simulink model "speedgoat_test_SN5659_R2021b"  (R2021b)
settings: Solver=FixedStepDiscrete  StartTime=0.0  StopTime=inf  RelTol=1e-3
PreLoadFcn:
  | Ts_IO107 = 0.001;
  | Ts_IO107 = 0.001;
  | Ts_IO133 = 0.001
  | 
  | Ts_IO204 = 0.001;
  | 
  | 
  | Ts_IO503 = 0.01;
  | 
  | ts_IO612 = 1e-3;
  | Ts_IO682 = 0.005;
  | Ts_IO941 = 0.01;
InitFcn:
  | Ts_IO107 = 0.001;
  | Ts_IO107 = 0.001;
  | Ts_IO133 = 0.001
  | 
  | Ts_IO204 = 0.001;
  | 
  | 
  | Ts_IO503 = 0.01;
  | 
  | ts_IO612 = 1e-3;
  | Ts_IO682 = 0.005;
  | Ts_IO941 = 0.01;
StopFcn:
  | if isfile(['sdi_view_',bdroot,'.mldatx'])
  |  Simulink.sdi.clearPreferences();
  |  Simulink.sdi.view();
  |  pause(3);
  |  Simulink.sdi.loadView(['sdi_view_',bdroot,]);
  | end
undefined symbols (not defined in the file): C, IO682, standard
libraries: speedgoatlib_IO682 x161, simulink x49, slrealtimeseriallib x16, canmsglib x12, speedgoatlib_serial x9, speedgoatlib_IO612 x9, speedgoatlib_IO133 x5, speedgoatlib_IO107 x4, speedgoatlib_IO204 x3, speedgoatlib_IO421 x3, speedgoatlib_PIL x1
(part 1 of 4)
settings Model: Creator=yannick.orgas  LastModifiedBy=ACH
settings SolverCC: ConcurrentTasks=on  AlgebraicLoopSolver=TrustRegion  PositivePriorityOrder=on
settings DataIOCC: LimitDataPoints=on  SaveFormat=StructureWithTime
settings OptimizationCC: BlockReduction=off  OptimizeBlockIOStorage=off
settings DebuggingCC: TasksWithSamePriorityMsg=none  UnconnectedInputMsg=none  UnconnectedOutputMsg=none  UnconnectedLineMsg=none  SFMachineParentedDataDiag=warning
settings HardwareCC: ProdBitPerLong=64  ProdLongLongMode=on  ProdHWDeviceType=Intel->x86-64 (Linux 64)
settings RTWCC: Description=Simulink Real-Time  SystemTargetFile=slrealtime.tlc  TemplateMakefile=slrealtime_default_tmf  Toolchain=Simulink Real-Time Toolchain  BuildConfiguration=Faster Runs  CodeExecutionProfiling=on  TargetLang=C++
settings SimulinkRealTimeTargetCC: UseGCCFastMath=on

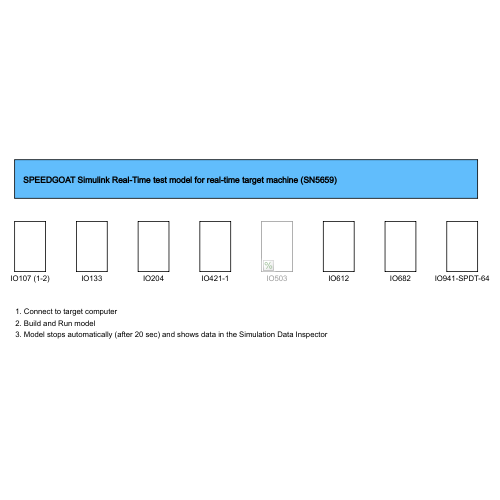
[thumbnail: Simulink's stored preview of the top-level diagram]
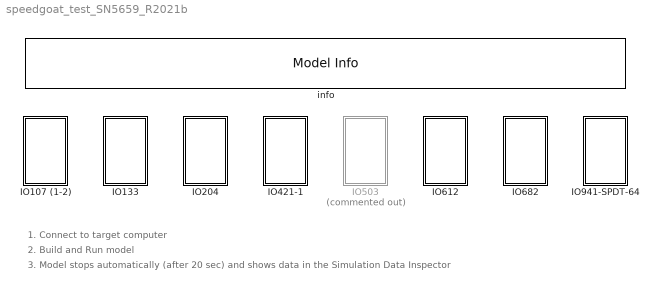
== system speedgoat_test_SN5659_R2021b ==
  note: 1. Connect to target computer
  note: 2. Build and Run model
  note: 3. Model stops automatically (after 20 sec) and shows data in the Simulation Data Inspector
  IO107 (1-2) : Subsystem
  IO133 : Subsystem
  IO204 : Subsystem
  IO421-1 : Subsystem
  IO503 : Subsystem  Commented=on
  IO612 : Subsystem
  IO682 : Subsystem
  IO941-SPDT-64 : Subsystem
  info : simulink/Model-Wide Utilities/Model Info  Frame=on  DisplayStringWithTags=SPEEDGOAT Simulink Real-Time test model for real-time target machine (SN5659)  HorizontalTextAlignment=Left  LeftAlignmentValue=0.02

== system speedgoat_test_SN5659_R2021b/IO107 (1-2) ==
  Analog output : speedgoatlib_IO107/Analog output  id=1  ts=-1  index=[1 2 3 4 5 6 7 8 9 10 11 12 13 14 15 16]  channels=[1 2 3 4 5 6 7 8 9 10 11 12 13 14 15 16]  range=1  pciSlot=-1
      settings: SourceProductName=Simulink Real-Time: Speedgoat Library
  Analog output1 : speedgoatlib_IO107/Analog output  id=2  ts=-1  index=[1 2 3 4 5 6 7 8 9 10 11 12 13 14 15 16]  channels=[1 2 3 4 5 6 7 8 9 10 11 12 13 14 15 16]  range=1  pciSlot=-1
      settings: SourceProductName=Simulink Real-Time: Speedgoat Library
  Setup : speedgoatlib_IO107/Setup  group=Analog output setup  id=1  range=+-10V  triggerSignal=TTL  groundSense=off  cal=on  pciSlot=-1  daChannel=[1:16]  daInitValue=[0]  daReset=[1]
      settings: SourceProductName=Simulink Real-Time: Speedgoat Library
  Setup1 : speedgoatlib_IO107/Setup  group=Module setup  id=2  range=+-10V  triggerSignal=TTL  groundSense=off  cal=on  pciSlot=-1  daChannel=[1:16]  daInitValue=[0]  daReset=[1]
      settings: SourceProductName=Simulink Real-Time: Speedgoat Library
  Sine Wave : Sin  Amplitude=10  Frequency=2*pi*50  SampleTime=Ts_IO107
  Sine Wave1 : Sin  Amplitude=10  Frequency=2*pi*50  SampleTime=Ts_IO107
  wires:
  Sine Wave/1 -> Analog output/1, Analog output/2, Analog output/3, Analog output/4, Analog output/5, Analog output/6, Analog output/7, Analog output/8, Analog output/9, Analog output/10, Analog output/11, Analog output/12, Analog output/13, Analog output/14, Analog output/15, Analog output/16
  Sine Wave1/1 -> Analog output1/1, Analog output1/2, Analog output1/3, Analog output1/4, Analog output1/5, Analog output1/6, Analog output1/7, Analog output1/8, Analog output1/9, Analog output1/10, Analog output1/11, Analog output1/12, Analog output1/13, Analog output1/14, Analog output1/15, Analog output1/16

== system speedgoat_test_SN5659_R2021b/IO133 ==
  "Analog input v2 " : speedgoatlib_IO133/Analog input v2   parModuleId=1  parSampleTime=Ts_IO133  parPciSlot=-1  parAdcChannels=[1 2 3 4]  parAdcVoltageRange=[2 2]  parAdcOversamplRate=[1 1]  parAdcContSampling=0  parAdcDmaEnable=0  parAdcActiveDmaDevices=[1 1]  parAdcFrameSize=100
      settings: SourceProductName=Simulink Real-Time: Speedgoat I/O Driver Library
  "Analog output v2 " : speedgoatlib_IO133/Analog output v2   parModuleId=1  parSampleTime=Ts_IO133  parPciSlot=-1  parDacChannels=[1 2 3 4]  parDacVoltageRange=[4 4 6 6 5 5 5 5]  parDacInitValues=[0 0 0 0]  parDacReset=[1 1 1 1]  parDacSyncOut=1  parDacDmaEnable=0  parDacActiveDmaDevices=[1 1]  parDacDmaLatency=2  parDacFrameSize=100
      settings: SourceProductName=Simulink Real-Time: Speedgoat I/O Driver Library
  "Digital input v2 " : speedgoatlib_IO133/Digital input v2   parModuleId=1  parSampleTime=Ts_IO133  parPciSlot=-1  parDiChannels=[8 9]
      settings: SourceProductName=Simulink Real-Time: Speedgoat I/O Driver Library
  "Digital output v2 " : speedgoatlib_IO133/Digital output v2   parModuleId=1  parSampleTime=Ts_IO133  parPciSlot=-1  parDoChannels=[1 2]  parDoInitValues=[0 0]  parDoReset=[1 1]
      settings: SourceProductName=Simulink Real-Time: Speedgoat I/O Driver Library
  Gain : Gain  Gain=2
  Gain1 : Gain  Gain=4
  Gain2 : Gain  Gain=6
  Gain3 : Gain  Gain=8
  Pulse Generator : DiscretePulseGenerator  Period=20  PulseWidth=5  SampleTime=Ts_IO133
  Pulse Generator1 : DiscretePulseGenerator  Period=20  PulseWidth=10  SampleTime=Ts_IO133
  "Scope 2 " : Scope  NumInputPorts=4
  "Scope 4 " : Scope  NumInputPorts=2
  "Setup v2 " : speedgoatlib_IO133/Setup v2   parPciSlot=-1  parModuleId=1  parInterModuleSync=None  parConvClockBaseRate=20MHz  parConvClock1Divider=20000  parConvClock2Divider=20000  parFrameTriggerEnable=off  parFrameTriggerDivider=10  parConvClock1BaseRate=1  parConvClock2BaseRate=1  parFrameTriggerClock=1  parAdcChannels=1:4  parAdcRange1=+-10V  parAdcRange2=+-10V  parAdcVoltageRange=[2 2]  parAdcOversampling1=None  parAdcOversampling2=None  parAdcOversamplRate=[1 1]  parAdcAutoCorrection=on  parAdcContSampling=off  parAdcDmaEnable=off  parAdcDmaClock=Clock 1  parAdcFrameSize_=100  parAdcSampleTime_=-1  parAdcActiveDmaDevices=[1 1]  parAdcFrameTriggerEnable=0  parAdcFrameSize=100  parAdcSampleTime=0.1  parDacChannels=1:4  parDacInitValues=0  parDacReset=1  parDacRange1=+-5V  parDacRange2=+-5V  parDacRange3=+-10.8V  parDacRange4=+-10.8V  parDacRange5=+-10V  parDacRange6=+-10V  parDacRange7=+-10V  parDacRange8=+-10V  parDacVoltageRange=[4 4 6 6 5 5 5 5]  parDacAutoCorrection=on  parDacSyncOut=on  parDacDmaEnable=off  parDacDmaLatency=Until next frame  parDacDmaClock=Clock 1  parDacFrameSize_=100  parDacSampleTime_=-1  parDacActiveDmaDevices=[1 1]  parDacFrameTriggerEnable=0  parDacFrameSize=100  parDacSampleTime=0.1  parDoChannels=1:2  parDoInitValues=0  parDoReset=1  parDiChannels=8:9  parDiDebounceEnable=off  parDiDebounceTime=0  parDiDebounceValue=0  parDioPullRefFront=Pull-up 3.3V  parDioPullRefRear=Floating
      settings: SourceProductName=Simulink Real-Time: Speedgoat I/O Driver Library
  Sine Wave : Sin  Frequency=50  SampleTime=0
  wires:
  Pulse Generator/1 -> "Digital output v2 "/1
  Gain1/1 -> "Analog output v2 "/2
  Gain/1 -> "Analog output v2 "/1
  Gain3/1 -> "Analog output v2 "/4
  Gain2/1 -> "Analog output v2 "/3
  Sine Wave/1 -> Gain/1, Gain1/1, Gain2/1, Gain3/1
  Pulse Generator1/1 -> "Digital output v2 "/2
  "Analog input v2 "/1 -> "Scope 2 "/1  "IO133_AI_CH1"
  "Analog input v2 "/2 -> "Scope 2 "/2  "IO133_AI_CH2"
  "Analog input v2 "/3 -> "Scope 2 "/3  "IO133_AI_CH3"
  "Analog input v2 "/4 -> "Scope 2 "/4  "IO133_AI_CH4"
  "Digital input v2 "/1 -> "Scope 4 "/1  "IO133_DI_CH8"
  "Digital input v2 "/2 -> "Scope 4 "/2  "IO133_DI_CH9"

== system speedgoat_test_SN5659_R2021b/IO204 ==
  Gain : Gain  Gain=2
  Gain1 : Gain  Gain=3
  Gain2 : Gain  Gain=4
  Pulse Generator : DiscretePulseGenerator  Period=20  PulseWidth=10  SampleTime=Ts_IO204
  Read : speedgoatlib_IO204/Read  id=1  group=Input  portType=16 ports of type double  ts=Ts_IO204  pciSlot=-1
      settings: SourceProductName=Simulink Real-Time: Speedgoat Library
  "Scope (xPC) " : Scope  NumInputPorts=4
  Setup : speedgoatlib_IO204/Setup  group=Module setup  id=1  pciSlot=-1  debounceEnable=on  debounceValue=0.001/10  reset=[0]  value=[0]
      settings: SourceProductName=Simulink Real-Time: Speedgoat Library
  Write : speedgoatlib_IO204/Write  id=1  portType=16 ports of type double  ts=-1  pciSlot=-1
      settings: SourceProductName=Simulink Real-Time: Speedgoat Library
  wires:
  Pulse Generator/1 -> Write/16, Write/11, Write/6, Write/1
  Read/6 -> Gain/1
  Read/11 -> Gain1/1
  Read/16 -> Gain2/1
  Read/1 -> "Scope (xPC) "/1  "IO204_CH1"
  Gain/1 -> "Scope (xPC) "/2  "IO204_CH6"
  Gain1/1 -> "Scope (xPC) "/3  "IO204_CH11"
  Gain2/1 -> "Scope (xPC) "/4  "IO204_CH16"

== system speedgoat_test_SN5659_R2021b/IO421-1 ==
  LVDT read : speedgoatlib_IO421/LVDT//RVDT/LVDT read  id=1  slot=1  channels=1  wiring=0  expectedVLL=7.0711  expectedVREF=18.3848  ts=0.001  pciSlot=-1
      settings: SourceProductName=Simulink Real-Time: Speedgoat Library
  LVDT read1 : speedgoatlib_IO421/LVDT//RVDT/LVDT read  id=1  slot=2  channels=1  wiring=0  expectedVLL=7.0711  expectedVREF=18.3848  ts=0.001  pciSlot=-1
      settings: SourceProductName=Simulink Real-Time: Speedgoat Library
  REF : speedgoatlib_IO421/W/REF  id=1  slot=3  frequency=47  voltage=26/sqrt(2)  pciSlot=-1
      settings: SourceProductName=Simulink Real-Time: Speedgoat I/O Blockset
  "Scope  " : Scope
  Scope  1 : Scope
  wires:
  LVDT read/1 -> "Scope  "/1  "IO421_LVDT_POS(1)"
  LVDT read1/1 -> Scope  1/1  "IO421_LVDT_POS(2)"

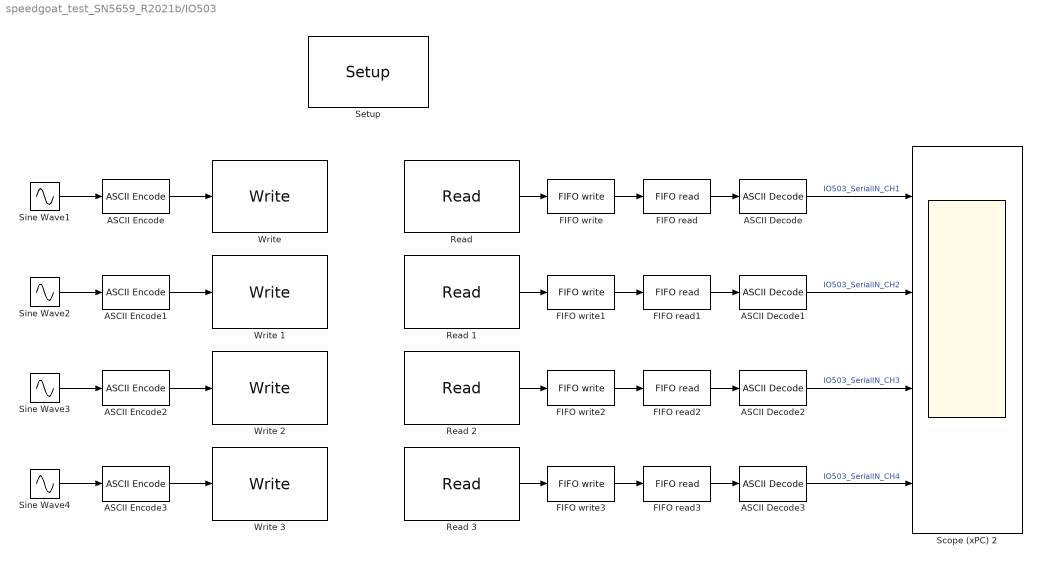
== system speedgoat_test_SN5659_R2021b/IO503 ==
  ASCII Decode{,1..3} (4 alike) : slrealtimeseriallib/ASCII Decode  format=%f\r  nvars=1  vartypes={'double'}
      settings: SourceProductBaseCode=XP
  ASCII Encode{,1..3} (4 alike) : slrealtimeseriallib/ASCII Encode  format=%f\r  nvars=1  maxlength=64  vartypes={ 'double' }
      settings: SourceProductBaseCode=XP
  FIFO read{,1..3} (4 alike) : slrealtimeseriallib/FIFO read  maxsize=64  minsize=1  usedelimiter=on  delimiter=13  outputtype=8 bit uint null terminated  enable=off  enableout=off  sampletime=Ts_IO503
      settings: SourceProductBaseCode=XP
  FIFO write : slrealtimeseriallib/FIFO write  size=64  inputtype=count+32 bit uint  present=off  sampletime=-1  id=Rx Ch1 overflow
      settings: SourceProductBaseCode=XP
  FIFO write1 : slrealtimeseriallib/FIFO write  size=64  inputtype=count+32 bit uint  present=off  sampletime=-1  id=Rx Ch2 overflow
      settings: SourceProductBaseCode=XP
  FIFO write2 : slrealtimeseriallib/FIFO write  size=64  inputtype=count+32 bit uint  present=off  sampletime=-1  id=Rx Ch3 overflow
      settings: SourceProductBaseCode=XP
  FIFO write3 : slrealtimeseriallib/FIFO write  size=64  inputtype=count+32 bit uint  present=off  sampletime=-1  id=Rx Ch4 overflow
      settings: SourceProductBaseCode=XP
  "Read " : speedgoatlib_serial/Speedgoat Shared blocks/Read   parModuleType=IO503  parModuleId=1  parChannel=1  parSampleTime=Ts_IO503  parFlush=on  parEnLegacy=on  parDataType=count+32 bit uint  parSlot=-1  parRxSwFifoSize=64
  Read 1 : speedgoatlib_serial/Speedgoat Shared blocks/Read   parModuleType=IO503  parModuleId=1  parChannel=2  parSampleTime=Ts_IO503  parFlush=on  parEnLegacy=on  parDataType=count+32 bit uint  parSlot=-1  parRxSwFifoSize=64
  Read 2 : speedgoatlib_serial/Speedgoat Shared blocks/Read   parModuleType=IO503  parModuleId=1  parChannel=3  parSampleTime=Ts_IO503  parFlush=on  parEnLegacy=on  parDataType=count+32 bit uint  parSlot=-1  parRxSwFifoSize=64
  Read 3 : speedgoatlib_serial/Speedgoat Shared blocks/Read   parModuleType=IO503  parModuleId=1  parChannel=4  parSampleTime=Ts_IO503  parFlush=on  parEnLegacy=on  parDataType=count+32 bit uint  parSlot=-1  parRxSwFifoSize=64
  "Scope (xPC) 2 " : Scope  NumInputPorts=4
  "Setup " : speedgoatlib_serial/Speedgoat Shared blocks/Setup   parModuleType=IO503  parModuleId=1  parSlot=-1  parTransceiver1=RS232  parTransceiver2=RS232  parTransceiver3=RS422  parTransceiver4=RS422  parTransceiver5=RS232  parTransceiver6=RS232  parTransceiver7=RS232  parTransceiver8=RS232  parTxTerm1=off  parRxTerm1=off  parMessageMonitoring1=off  parAutoTurnaround1=off  parTurnaroundDelay1=0  parStandardBaud1=on  parBaudrate1=921600  parBaudDivisor1=1  parSamplingRate1=16x (standard)  parPrescale1=off  parCalcBaud1=2764800  parParity1=None  parDataBits1=8  parStopBits1=1  parTxTrigLvl1=1  parRxTrigLvl1=8  parHandshake1=none  parRtsHysteresis1=0  parXon1=17  parXoff1=19  parTxSwFifoSize1=64  parRxSwFifoSize1=64  parTxTerm2=off  parRxTerm2=off  parMessageMonitoring2=off  parAutoTurnaround2=off  parTurnaroundDelay2=0  parStandardBaud2=on  parBaudrate2=921600  parBaudDivisor2=1  parSamplingRate2=16x (standard)  parPrescale2=off  parCalcBaud2=2764800  parParity2=None  parDataBits2=8  parStopBits2=1  parTxTrigLvl2=1  parRxTrigLvl2=8  parHandshake2=none  parRtsHysteresis2=0  parXon2=17  parXoff2=19  parTxSwFifoSize2=64  parRxSwFifoSize2=64  parTxTerm3=off  parRxTerm3=on  parMessageMonitoring3=off  parAutoTurnaround3=off  parTurnaroundDelay3=0  parStandardBaud3=on  parBaudrate3=2764800  parBaudDivisor3=1  parSamplingRate3=16x (standard)  parPrescale3=off  parCalcBaud3=2764800  parParity3=None  parDataBits3=8  parStopBits3=1  parTxTrigLvl3=1  parRxTrigLvl3=8  parHandshake3=none  parRtsHysteresis3=0  parXon3=17  parXoff3=19  parTxSwFifoSize3=64  parRxSwFifoSize3=64  parTxTerm4=off  parRxTerm4=on  parMessageMonitoring4=off  parAutoTurnaround4=off  parTurnaroundDelay4=0  parStandardBaud4=on  parBaudrate4=2764800  parBaudDivisor4=1  parSamplingRate4=16x (standard)  parPrescale4=off  parCalcBaud4=2764800  parParity4=None  parDataBits4=8  parStopBits4=1  parTxTrigLvl4=1  parRxTrigLvl4=8  parHandshake4=none  parRtsHysteresis4=0  parXon4=17  parXoff4=19  parTxSwFifoSize4=64  parRxSwFifoSize4=64  parTxTerm5=off  parRxTerm5=off  parMessageMonitoring5=off  parAutoTurnaround5=off  parTurnaroundDelay5=0  parStandardBaud5=on  parBaudrate5=115200  parBaudDivisor5=1  parSamplingRate5=16x (standard)  parPrescale5=off  parCalcBaud5=2764800  parParity5=None  parDataBits5=8  parStopBits5=1  parTxTrigLvl5=1  parRxTrigLvl5=1  parHandshake5=none  parRtsHysteresis5=0  parXon5=17  parXoff5=19  parTxSwFifoSize5=1024  parRxSwFifoSize5=1024  parTxTerm6=off  parRxTerm6=off  parMessageMonitoring6=off  parAutoTurnaround6=off  parTurnaroundDelay6=0  parStandardBaud6=on  parBaudrate6=115200  parBaudDivisor6=1  parSamplingRate6=16x (standard)  parPrescale6=off  parCalcBaud6=2764800  parParity6=None  parDataBits6=8  parStopBits6=1  parTxTrigLvl6=1  parRxTrigLvl6=1  parHandshake6=none  parRtsHysteresis6=0  parXon6=17  parXoff6=19  parTxSwFifoSize6=1024  parRxSwFifoSize6=1024  parTxTerm7=off  parRxTerm7=off  parMessageMonitoring7=off  parAutoTurnaround7=off  parTurnaroundDelay7=0  parStandardBaud7=on  parBaudrate7=115200  parBaudDivisor7=1  parSamplingRate7=16x (standard)  parPrescale7=off  parCalcBaud7=2764800  parParity7=None  parDataBits7=8  parStopBits7=1  parTxTrigLvl7=1  parRxTrigLvl7=1  parHandshake7=none  parRtsHysteresis7=0  parXon7=17  parXoff7=19  parTxSwFifoSize7=1024  parRxSwFifoSize7=1024  parTxTerm8=off  parRxTerm8=off  parMessageMonitoring8=off  parAutoTurnaround8=off  parTurnaroundDelay8=0  parStandardBaud8=on  parBaudrate8=115200  parBaudDivisor8=1  parSamplingRate8=16x (standard)  parPrescale8=off  parCalcBaud8=2764800  parParity8=None  parDataBits8=8  parStopBits8=1  parTxTrigLvl8=1  parRxTrigLvl8=1  parHandshake8=none  parRtsHysteresis8=0  parXon8=17  parXoff8=19  parTxSwFifoSize8=1024  parRxSwFifoSize8=1024
      settings: SourceProductName=Simulink Real-Time: Speedgoat I/O Driver Library
  Sine Wave1 : Sin  Amplitude=10  Bias=127  Frequency=1*2*pi  SampleTime=Ts_IO503
  Sine Wave2 : Sin  Amplitude=20  Bias=127  Frequency=1*2*pi  SampleTime=Ts_IO503
  Sine Wave3 : Sin  Amplitude=30  Bias=127  Frequency=1*2*pi  SampleTime=Ts_IO503
  Sine Wave4 : Sin  Amplitude=40  Bias=127  Frequency=1*2*pi  SampleTime=Ts_IO503
  "Write " : speedgoatlib_serial/Speedgoat Shared blocks/Write   parModuleType=IO503  parModuleId=1  parChannel=1  parSampleTime=-1  parEnLegacy=on  parDataType=8 bit uint null terminated  parSlot=-1  parTxSwFifoSize=64
  Write 1 : speedgoatlib_serial/Speedgoat Shared blocks/Write   parModuleType=IO503  parModuleId=1  parChannel=2  parSampleTime=-1  parEnLegacy=on  parDataType=8 bit uint null terminated  parSlot=-1  parTxSwFifoSize=64
  Write 2 : speedgoatlib_serial/Speedgoat Shared blocks/Write   parModuleType=IO503  parModuleId=1  parChannel=3  parSampleTime=-1  parEnLegacy=on  parDataType=8 bit uint null terminated  parSlot=-1  parTxSwFifoSize=64
  Write 3 : speedgoatlib_serial/Speedgoat Shared blocks/Write   parModuleType=IO503  parModuleId=1  parChannel=4  parSampleTime=-1  parEnLegacy=on  parDataType=8 bit uint null terminated  parSlot=-1  parTxSwFifoSize=64
  wires:
  Sine Wave4/1 -> ASCII Encode3/1
  Sine Wave3/1 -> ASCII Encode2/1
  Sine Wave1/1 -> ASCII Encode/1
  Sine Wave2/1 -> ASCII Encode1/1
  ASCII Decode/1 -> "Scope (xPC) 2 "/1  "IO503_SerialIN_CH1"
  ASCII Decode1/1 -> "Scope (xPC) 2 "/2  "IO503_SerialIN_CH2"
  ASCII Decode2/1 -> "Scope (xPC) 2 "/3  "IO503_SerialIN_CH3"
  ASCII Decode3/1 -> "Scope (xPC) 2 "/4  "IO503_SerialIN_CH4"
  FIFO write/1 -> FIFO read/1
  "Read "/1 -> FIFO write/1
  FIFO write1/1 -> FIFO read1/1
  Read 1/1 -> FIFO write1/1
  FIFO write2/1 -> FIFO read2/1
  FIFO write3/1 -> FIFO read3/1
  FIFO read1/1 -> ASCII Decode1/1
  FIFO read2/1 -> ASCII Decode2/1
  FIFO read3/1 -> ASCII Decode3/1
  Read 2/1 -> FIFO write2/1
  Read 3/1 -> FIFO write3/1
  ASCII Encode/1 -> "Write "/1
  FIFO read/1 -> ASCII Decode/1
  ASCII Encode1/1 -> Write 1/1
  ASCII Encode2/1 -> Write 2/1
  ASCII Encode3/1 -> Write 3/1

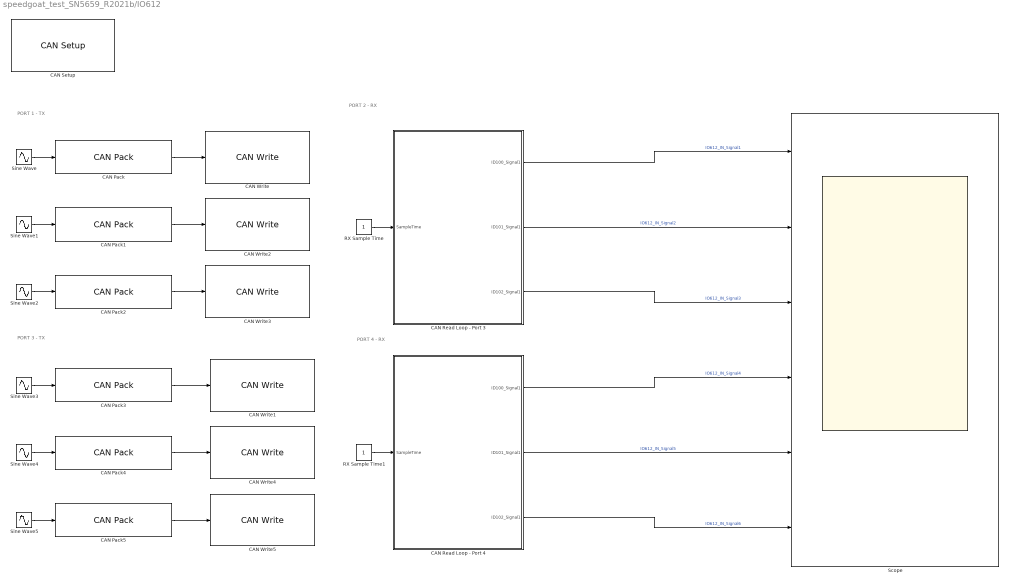
== system speedgoat_test_SN5659_R2021b/IO612 ==
  note: PORT 4 - RX
  note: PORT 1 - TX
  note: PORT 3 - TX
  note: PORT 2 - RX
  CAN Pack : canmsglib/CAN Pack  MsgList=(none)  MsgName=CAN Msg  MsgIDType=Standard (11-bit identifier)  MsgIdentifier=100  MsgLength=8  Remote=off  ApplyMinMax=off  BusOutput=off  SignalInfo={'Signal1','0','64','LE','double','Standard','0','1','0','-Inf','Inf'}
      settings: SourceProductBaseCode=ME,XP,VN  DataFormat=manually specified signals
  CAN Pack1 : canmsglib/CAN Pack  MsgList=(none)  MsgName=CAN Msg  MsgIDType=Standard (11-bit identifier)  MsgIdentifier=101  MsgLength=8  Remote=off  ApplyMinMax=off  BusOutput=off  SignalInfo={'Signal1','0','64','LE','double','Standard','0','1','0','-Inf','Inf'}
      settings: SourceProductBaseCode=ME,XP,VN  DataFormat=manually specified signals
  CAN Pack2 : canmsglib/CAN Pack  MsgList=(none)  MsgName=CAN Msg  MsgIDType=Standard (11-bit identifier)  MsgIdentifier=102  MsgLength=8  Remote=off  ApplyMinMax=off  BusOutput=off  SignalInfo={'Signal1','0','64','LE','double','Standard','0','1','0','-Inf','Inf'}
      settings: SourceProductBaseCode=ME,XP,VN  DataFormat=manually specified signals
  CAN Pack3 : canmsglib/CAN Pack  MsgList=(none)  MsgName=CAN Msg  MsgIDType=Standard (11-bit identifier)  MsgIdentifier=300  MsgLength=8  Remote=off  ApplyMinMax=off  BusOutput=off  SignalInfo={'Signal1','0','64','LE','double','Standard','0','1','0','-Inf','Inf'}
      settings: SourceProductBaseCode=ME,XP,VN  DataFormat=manually specified signals
  CAN Pack4 : canmsglib/CAN Pack  MsgList=(none)  MsgName=CAN Msg  MsgIDType=Standard (11-bit identifier)  MsgIdentifier=301  MsgLength=8  Remote=off  ApplyMinMax=off  BusOutput=off  SignalInfo={'Signal1','0','64','LE','double','Standard','0','1','0','-Inf','Inf'}
      settings: SourceProductBaseCode=ME,XP,VN  DataFormat=manually specified signals
  CAN Pack5 : canmsglib/CAN Pack  MsgList=(none)  MsgName=CAN Msg  MsgIDType=Standard (11-bit identifier)  MsgIdentifier=302  MsgLength=8  Remote=off  ApplyMinMax=off  BusOutput=off  SignalInfo={'Signal1','0','64','LE','double','Standard','0','1','0','-Inf','Inf'}
      settings: SourceProductBaseCode=ME,XP,VN  DataFormat=manually specified signals
  CAN Read Loop - Port 3 : Subsystem  TreatAsAtomicUnit=on
  CAN Read Loop - Port 4 : Subsystem  TreatAsAtomicUnit=on
  CAN Setup : speedgoatlib_IO612/CAN Setup  id=1  drvLtr=C:  PCISlot=-1  port1=CAN (HS)  port2=CAN (HS)  port3=CAN (HS)  port4=CAN (HS)  opModeCAN1=Highspeed (HS)  bdrCAN1=1 MBaud  usrBdrCAN1=[5, 1, 13, 2]  stdAccMaskCAN1=[0, 0]  extAccMaskCAN1=[0, 0]  opModeCAN2=Highspeed (HS)  bdrCAN2=1 MBaud  usrBdrCAN2=[5, 1, 13, 2]  stdAccMaskCAN2=[0, 0]  extAccMaskCAN2=[0, 0]  opModeCAN3=Highspeed (HS)  bdrCAN3=1 MBaud  usrBdrCAN3=[5, 1, 13, 2]  stdAccMaskCAN3=[0, 0]  extAccMaskCAN3=[0, 0]  opModeCAN4=Highspeed (HS)  bdrCAN4=1 MBaud  usrBdrCAN4=[5, 1, 13, 2]  stdAccMaskCAN4=[0, 0]  extAccMaskCAN4=[0, 0]  initStruct=[]  termStruct=[]  protl=IO612  qtyMod=1  chNo=[1, 2, 3, 4]  ptTypes=[1, 1, 1, 1]  protlHelpIdx=[0, 1, 2, 3]  isFDMod=0
      settings: SourceProductName=Simulink Real-Time: Speedgoat Library
  CAN Write : speedgoatlib_IO612/CAN Write  id=1  sampleTime=ts_IO612  portSelection=1  messageType=CAN  BusInput=off  enaStatusPort=off  protl=IO612  ptIdx=0  isFDMod=0
      settings: SourceProductName=Simulink Real-Time: Speedgoat Library
  CAN Write1 : speedgoatlib_IO612/CAN Write  id=1  sampleTime=ts_IO612  portSelection=3  messageType=CAN  BusInput=off  enaStatusPort=off  protl=IO612  ptIdx=2  isFDMod=0
      settings: SourceProductName=Simulink Real-Time: Speedgoat Library
  CAN Write2 : speedgoatlib_IO612/CAN Write  id=1  sampleTime=ts_IO612  portSelection=1  messageType=CAN  BusInput=off  enaStatusPort=off  protl=IO612  ptIdx=0  isFDMod=0
      settings: SourceProductName=Simulink Real-Time: Speedgoat Library
  CAN Write3 : speedgoatlib_IO612/CAN Write  id=1  sampleTime=ts_IO612  portSelection=1  messageType=CAN  BusInput=off  enaStatusPort=off  protl=IO612  ptIdx=0  isFDMod=0
      settings: SourceProductName=Simulink Real-Time: Speedgoat Library
  CAN Write4 : speedgoatlib_IO612/CAN Write  id=1  sampleTime=ts_IO612  portSelection=3  messageType=CAN  BusInput=off  enaStatusPort=off  protl=IO612  ptIdx=2  isFDMod=0
      settings: SourceProductName=Simulink Real-Time: Speedgoat Library
  CAN Write5 : speedgoatlib_IO612/CAN Write  id=1  sampleTime=ts_IO612  portSelection=3  messageType=CAN  BusInput=off  enaStatusPort=off  protl=IO612  ptIdx=2  isFDMod=0
      settings: SourceProductName=Simulink Real-Time: Speedgoat Library
  RX Sample Time : Constant  SampleTime=ts_IO612
  RX Sample Time1 : Constant  SampleTime=ts_IO612
  "Scope  " : Scope  NumInputPorts=6
  Sine Wave : Sin  Amplitude=10  Frequency=2*pi*10  SampleTime=ts_IO612
  Sine Wave1 : Sin  Amplitude=20  Frequency=2*pi*10  SampleTime=ts_IO612
  Sine Wave2 : Sin  Amplitude=30  Frequency=2*pi*10  SampleTime=ts_IO612
  Sine Wave3 : Sin  Amplitude=40  Frequency=2*pi*10  SampleTime=ts_IO612
  Sine Wave4 : Sin  Amplitude=50  Frequency=2*pi*10  SampleTime=ts_IO612
  Sine Wave5 : Sin  Amplitude=60  Frequency=2*pi*10  SampleTime=ts_IO612
  wires:
  RX Sample Time1/1 -> CAN Read Loop - Port 4/1(SampleTime)
  CAN Pack4/1 -> CAN Write4/1
  RX Sample Time/1 -> CAN Read Loop - Port 3/1(SampleTime)
  CAN Pack3/1 -> CAN Write1/1
  Sine Wave1/1 -> CAN Pack1/1
  Sine Wave4/1 -> CAN Pack4/1
  Sine Wave3/1 -> CAN Pack3/1
  Sine Wave5/1 -> CAN Pack5/1
  Sine Wave/1 -> CAN Pack/1
  Sine Wave2/1 -> CAN Pack2/1
  CAN Pack5/1 -> CAN Write5/1
  CAN Pack/1 -> CAN Write/1
  CAN Pack1/1 -> CAN Write2/1
  CAN Pack2/1 -> CAN Write3/1
  CAN Read Loop - Port 3/1(ID100_Signal1) -> "Scope  "/1  "IO612_IN_Signal1"
  CAN Read Loop - Port 3/2(ID101_Signal1) -> "Scope  "/2  "IO612_IN_Signal2"
  CAN Read Loop - Port 3/3(ID102_Signal1) -> "Scope  "/3  "IO612_IN_Signal3"
  CAN Read Loop - Port 4/1(ID100_Signal1) -> "Scope  "/4  "IO612_IN_Signal4"
  CAN Read Loop - Port 4/2(ID101_Signal1) -> "Scope  "/5  "IO612_IN_Signal5"
  CAN Read Loop - Port 4/3(ID102_Signal1) -> "Scope  "/6  "IO612_IN_Signal6"

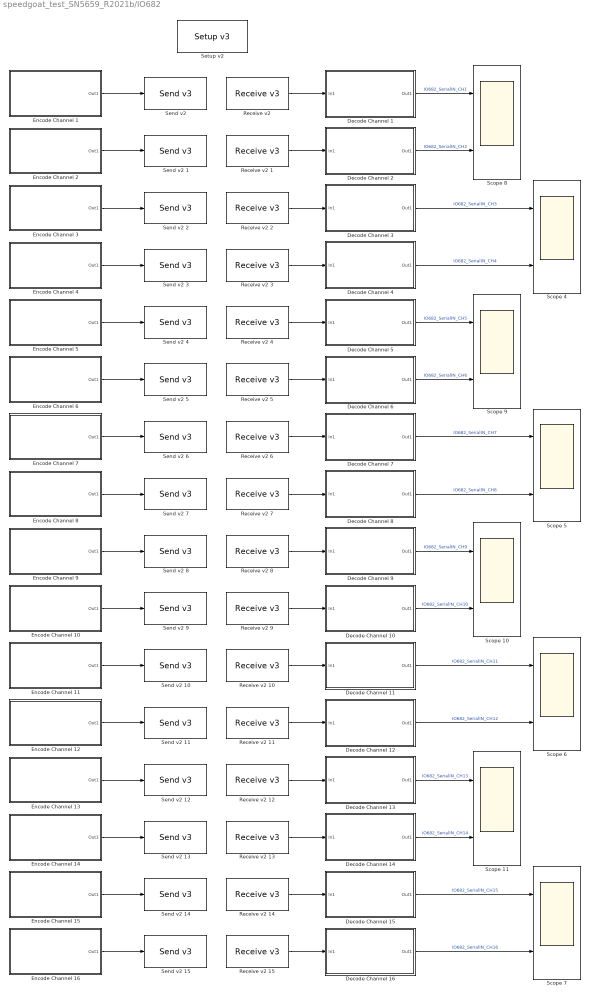
== system speedgoat_test_SN5659_R2021b/IO682 ==
  Decode Channel 1 : Subsystem
  Decode Channel 10 : Subsystem
  Decode Channel 11 : Subsystem
  Decode Channel 12 : Subsystem
  Decode Channel 13 : Subsystem
  Decode Channel 14 : Subsystem
  Decode Channel 15 : Subsystem
  Decode Channel 16 : Subsystem
  Decode Channel 2 : Subsystem
  Decode Channel 3 : Subsystem
  Decode Channel 4 : Subsystem
  Decode Channel 5 : Subsystem
  Decode Channel 6 : Subsystem
  Decode Channel 7 : Subsystem
  Decode Channel 8 : Subsystem
  Decode Channel 9 : Subsystem
  Encode Channel 1 : Subsystem
  Encode Channel 10 : Subsystem
  Encode Channel 11 : Subsystem
  Encode Channel 12 : Subsystem
  Encode Channel 13 : Subsystem
  Encode Channel 14 : Subsystem
  Encode Channel 15 : Subsystem
  Encode Channel 16 : Subsystem
  Encode Channel 2 : Subsystem
  Encode Channel 3 : Subsystem
  Encode Channel 4 : Subsystem
  Encode Channel 5 : Subsystem
  Encode Channel 6 : Subsystem
  Encode Channel 7 : Subsystem
  Encode Channel 8 : Subsystem
  Encode Channel 9 : Subsystem
  "Receive v2 " : speedgoatlib_IO682/Receive v3   parModuleId=1  parChannel=1  parMaxWords=50  parMinWords=1  parSampleTime=Ts_IO682
      settings: SourceProductName=Speedgoat I/O Blockset
  Receive v2 1 : speedgoatlib_IO682/Receive v3   parModuleId=1  parChannel=2  parMaxWords=50  parMinWords=1  parSampleTime=Ts_IO682
      settings: SourceProductName=Speedgoat I/O Blockset
  Receive v2 10 : speedgoatlib_IO682/Receive v3   parModuleId=1  parChannel=11  parMaxWords=50  parMinWords=1  parSampleTime=Ts_IO682
      settings: SourceProductName=Speedgoat I/O Blockset
  Receive v2 11 : speedgoatlib_IO682/Receive v3   parModuleId=1  parChannel=12  parMaxWords=50  parMinWords=1  parSampleTime=Ts_IO682
      settings: SourceProductName=Speedgoat I/O Blockset
  Receive v2 12 : speedgoatlib_IO682/Receive v3   parModuleId=1  parChannel=13  parMaxWords=50  parMinWords=1  parSampleTime=Ts_IO682
      settings: SourceProductName=Speedgoat I/O Blockset
  Receive v2 13 : speedgoatlib_IO682/Receive v3   parModuleId=1  parChannel=14  parMaxWords=50  parMinWords=1  parSampleTime=Ts_IO682
      settings: SourceProductName=Speedgoat I/O Blockset
  Receive v2 14 : speedgoatlib_IO682/Receive v3   parModuleId=1  parChannel=15  parMaxWords=50  parMinWords=1  parSampleTime=Ts_IO682
      settings: SourceProductName=Speedgoat I/O Blockset
  Receive v2 15 : speedgoatlib_IO682/Receive v3   parModuleId=1  parChannel=16  parMaxWords=50  parMinWords=1  parSampleTime=Ts_IO682
      settings: SourceProductName=Speedgoat I/O Blockset
  Receive v2 2 : speedgoatlib_IO682/Receive v3   parModuleId=1  parChannel=3  parMaxWords=50  parMinWords=1  parSampleTime=Ts_IO682
      settings: SourceProductName=Speedgoat I/O Blockset
  Receive v2 3 : speedgoatlib_IO682/Receive v3   parModuleId=1  parChannel=4  parMaxWords=50  parMinWords=1  parSampleTime=Ts_IO682
      settings: SourceProductName=Speedgoat I/O Blockset
  Receive v2 4 : speedgoatlib_IO682/Receive v3   parModuleId=1  parChannel=5  parMaxWords=50  parMinWords=1  parSampleTime=Ts_IO682
      settings: SourceProductName=Speedgoat I/O Blockset
  Receive v2 5 : speedgoatlib_IO682/Receive v3   parModuleId=1  parChannel=6  parMaxWords=50  parMinWords=1  parSampleTime=Ts_IO682
      settings: SourceProductName=Speedgoat I/O Blockset
  Receive v2 6 : speedgoatlib_IO682/Receive v3   parModuleId=1  parChannel=7  parMaxWords=50  parMinWords=1  parSampleTime=Ts_IO682
      settings: SourceProductName=Speedgoat I/O Blockset
  Receive v2 7 : speedgoatlib_IO682/Receive v3   parModuleId=1  parChannel=8  parMaxWords=50  parMinWords=1  parSampleTime=Ts_IO682
      settings: SourceProductName=Speedgoat I/O Blockset
  Receive v2 8 : speedgoatlib_IO682/Receive v3   parModuleId=1  parChannel=9  parMaxWords=50  parMinWords=1  parSampleTime=Ts_IO682
      settings: SourceProductName=Speedgoat I/O Blockset
  Receive v2 9 : speedgoatlib_IO682/Receive v3   parModuleId=1  parChannel=10  parMaxWords=50  parMinWords=1  parSampleTime=Ts_IO682
      settings: SourceProductName=Speedgoat I/O Blockset
  Scope {4..11} (8 alike) : Scope  NumInputPorts=2
  "Send v2 " : speedgoatlib_IO682/Send v3   parModuleId=1  parChannel=1  parSampleTime=Ts_IO682
      settings: SourceProductName=Speedgoat I/O Blockset
  Send v2 1 : speedgoatlib_IO682/Send v3   parModuleId=1  parChannel=2  parSampleTime=Ts_IO682
      settings: SourceProductName=Speedgoat I/O Blockset
  Send v2 10 : speedgoatlib_IO682/Send v3   parModuleId=1  parChannel=11  parSampleTime=Ts_IO682
      settings: SourceProductName=Speedgoat I/O Blockset
  Send v2 11 : speedgoatlib_IO682/Send v3   parModuleId=1  parChannel=12  parSampleTime=Ts_IO682
      settings: SourceProductName=Speedgoat I/O Blockset
  Send v2 12 : speedgoatlib_IO682/Send v3   parModuleId=1  parChannel=13  parSampleTime=Ts_IO682
      settings: SourceProductName=Speedgoat I/O Blockset
  Send v2 13 : speedgoatlib_IO682/Send v3   parModuleId=1  parChannel=14  parSampleTime=Ts_IO682
      settings: SourceProductName=Speedgoat I/O Blockset
  Send v2 14 : speedgoatlib_IO682/Send v3   parModuleId=1  parChannel=15  parSampleTime=Ts_IO682
      settings: SourceProductName=Speedgoat I/O Blockset
  Send v2 15 : speedgoatlib_IO682/Send v3   parModuleId=1  parChannel=16  parSampleTime=Ts_IO682
      settings: SourceProductName=Speedgoat I/O Blockset
  Send v2 2 : speedgoatlib_IO682/Send v3   parModuleId=1  parChannel=3  parSampleTime=Ts_IO682
      settings: SourceProductName=Speedgoat I/O Blockset
  Send v2 3 : speedgoatlib_IO682/Send v3   parModuleId=1  parChannel=4  parSampleTime=Ts_IO682
      settings: SourceProductName=Speedgoat I/O Blockset
  Send v2 4 : speedgoatlib_IO682/Send v3   parModuleId=1  parChannel=5  parSampleTime=Ts_IO682
      settings: SourceProductName=Speedgoat I/O Blockset
  Send v2 5 : speedgoatlib_IO682/Send v3   parModuleId=1  parChannel=6  parSampleTime=Ts_IO682
      settings: SourceProductName=Speedgoat I/O Blockset
  Send v2 6 : speedgoatlib_IO682/Send v3   parModuleId=1  parChannel=7  parSampleTime=Ts_IO682
      settings: SourceProductName=Speedgoat I/O Blockset
  Send v2 7 : speedgoatlib_IO682/Send v3   parModuleId=1  parChannel=8  parSampleTime=Ts_IO682
      settings: SourceProductName=Speedgoat I/O Blockset
  Send v2 8 : speedgoatlib_IO682/Send v3   parModuleId=1  parChannel=9  parSampleTime=Ts_IO682
      settings: SourceProductName=Speedgoat I/O Blockset
  Send v2 9 : speedgoatlib_IO682/Send v3   parModuleId=1  parChannel=10  parSampleTime=Ts_IO682
      settings: SourceProductName=Speedgoat I/O Blockset
  "Setup v2 " : speedgoatlib_IO682/Setup v3   parModuleId=1  parBoardVariant=IO682-16-16  parPciSlot=-1  parTimerCount=4000  parChannelMode=Manual  parInBitRate1=100000  parInBufferMode1=Individual  parInEnable1=on  parInParity1=on  parInInternalWrap1=off  parInBitRate2=100000  parInBufferMode2=Individual  parInEnable2=on  parInParity2=on  parInInternalWrap2=off  parInBitRate3=100000  parInBufferMode3=Individual  parInEnable3=on  parInParity3=on  parInInternalWrap3=off  parInBitRate4=100000  parInBufferMode4=Individual  parInEnable4=on  parInParity4=on  parInInternalWrap4=off  parInBitRate5=100000  parInBufferMode5=Individual  parInEnable5=on  parInParity5=on  parInInternalWrap5=off  parInBitRate6=100000  parInBufferMode6=Individual  parInEnable6=on  parInParity6=on  parInInternalWrap6=off  parInBitRate7=100000  parInBufferMode7=Individual  parInEnable7=on  parInParity7=on  parInInternalWrap7=off  parInBitRate8=100000  parInBufferMode8=Individual  parInEnable8=on  parInParity8=on  parInInternalWrap8=off  parInBitRate9=100000  parInBufferMode9=Individual  parInEnable9=on  parInParity9=on  parInInternalWrap9=off  parInBitRate10=100000  parInBufferMode10=Individual  parInEnable10=on  parInParity10=on  parInInternalWrap10=off  parInBitRate11=100000  parInBufferMode11=Individual  parInEnable11=on  parInParity11=on  parInInternalWrap11=off  parInBitRate12=100000  parInBufferMode12=Individual  parInEnable12=on  parInParity12=on  parInInternalWrap12=off  parInBitRate13=100000  parInBufferMode13=Individual  parInEnable13=on  parInParity13=on  parInInternalWrap13=off  parInBitRate14=100000  parInBufferMode14=Individual  parInEnable14=on  parInParity14=on  parInInternalWrap14=off  parInBitRate15=100000  parInBufferMode15=Individual  parInEnable15=on  parInParity15=on  parInInternalWrap15=off  parInBitRate16=100000  parInBufferMode16=Individual  parInEnable16=on  parInParity16=on  parInInternalWrap16=off  parOutBitRate1=100000  parOutParity1=Odd  parOutProtocolError1=None  parOutEnable1=on  parOutBitRate2=100000  parOutParity2=Odd  parOutProtocolError2=None  parOutEnable2=on  parOutBitRate3=100000  parOutParity3=Odd  parOutProtocolError3=None  parOutEnable3=on  parOutBitRate4=100000  parOutParity4=Odd  parOutProtocolError4=None  parOutEnable4=on  parOutBitRate5=100000  parOutParity5=Odd  parOutProtocolError5=None  parOutEnable5=on  parOutBitRate6=100000  parOutParity6=Odd  parOutProtocolError6=None  parOutEnable6=on  parOutBitRate7=100000  parOutParity7=Odd  parOutProtocolError7=None  parOutEnable7=on  parOutBitRate8=100000  parOutParity8=Odd  parOutProtocolError8=None  parOutEnable8=on  parOutBitRate9=100000  parOutParity9=Odd  parOutProtocolError9=None  parOutEnable9=on  parOutBitRate10=100000  parOutParity10=Odd  parOutProtocolError10=None  parOutEnable10=on  parOutBitRate11=100000  parOutParity11=Odd  parOutProtocolError11=None  parOutEnable11=on  parOutBitRate12=100000  parOutParity12=Odd  parOutProtocolError12=None  parOutEnable12=on  parOutBitRate13=100000  parOutParity13=Odd  parOutProtocolError13=None  parOutEnable13=on  parOutBitRate14=100000  parOutParity14=Odd  parOutProtocolError14=None  parOutEnable14=on  parOutBitRate15=100000  parOutParity15=Odd  parOutProtocolError15=None  parOutEnable15=on  parOutBitRate16=100000  parOutParity16=Odd  parOutProtocolError16=None  parOutEnable16=on  parChConfigFile=''  parScheduleMode=Manual  parScheduledMsgConfigFile=''  parHwDeviceId=hex2dec('0830')  parTimeSource=Internal timer  parChInConfig=[158 8 7 7 1;158 8 7 7 1;158 8 7 7 1;158 8 7 7 1;158 8 7 7 1;158 8 7 7 1;158 8 7 7 1;158 8 7 7 1;158 8 7 7 1;158 8 7 7 1;158 8 7 7 1;158 8 7 7 1;158 8 7 7 1;158 8 7 7 1;158 8 7 7 1;158 8 7 7 1]  parChOutConfig=[158 0 4 7;158 0 4 7;158 0 4 7;158 0 4 7;158 0 4 7;158 0 4 7;158 0 4 7;158 0 4 7;158 0 4 7;158 0 4 7;158 0 4 7;158 0 4 7;158 0 4 7;158 0 4 7;158 0 4 7;158 0 4 7]  parScheduledMessages=0
      settings: SourceProductName=Speedgoat I/O Blockset
  wires:
  Receive v2 3/1 -> Decode Channel 4/1(In1)
  Decode Channel 15/1(Out1) -> Scope 7/1  "IO682_SerialIN_CH15"
  "Receive v2 "/1 -> Decode Channel 1/1(In1)
  Receive v2 13/1 -> Decode Channel 14/1(In1)
  Decode Channel 11/1(Out1) -> Scope 6/1  "IO682_SerialIN_CH11"
  Encode Channel 15/1(Out1) -> Send v2 14/1
  Receive v2 8/1 -> Decode Channel 9/1(In1)
  Decode Channel 16/1(Out1) -> Scope 7/2  "IO682_SerialIN_CH16"
  Receive v2 15/1 -> Decode Channel 16/1(In1)
  Encode Channel 13/1(Out1) -> Send v2 12/1
  Encode Channel 14/1(Out1) -> Send v2 13/1
  Decode Channel 12/1(Out1) -> Scope 6/2  "IO682_SerialIN_CH12"
  Decode Channel 3/1(Out1) -> Scope 4/1  "IO682_SerialIN_CH3"
  Receive v2 14/1 -> Decode Channel 15/1(In1)
  Encode Channel 1/1(Out1) -> "Send v2 "/1
  Decode Channel 5/1(Out1) -> Scope 9/1  "IO682_SerialIN_CH5"
  Encode Channel 7/1(Out1) -> Send v2 6/1
  Receive v2 7/1 -> Decode Channel 8/1(In1)
  Decode Channel 14/1(Out1) -> Scope 11/2  "IO682_SerialIN_CH14"
  Decode Channel 10/1(Out1) -> Scope 10/2  "IO682_SerialIN_CH10"
  Encode Channel 9/1(Out1) -> Send v2 8/1
  Receive v2 2/1 -> Decode Channel 3/1(In1)
  Receive v2 10/1 -> Decode Channel 11/1(In1)
  Decode Channel 8/1(Out1) -> Scope 5/2  "IO682_SerialIN_CH8"
  Encode Channel 4/1(Out1) -> Send v2 3/1
  Encode Channel 6/1(Out1) -> Send v2 5/1
  Encode Channel 2/1(Out1) -> Send v2 1/1
  Receive v2 9/1 -> Decode Channel 10/1(In1)
  Encode Channel 16/1(Out1) -> Send v2 15/1
  Decode Channel 9/1(Out1) -> Scope 10/1  "IO682_SerialIN_CH9"
  Receive v2 11/1 -> Decode Channel 12/1(In1)
  Encode Channel 11/1(Out1) -> Send v2 10/1
  Encode Channel 10/1(Out1) -> Send v2 9/1
  Receive v2 12/1 -> Decode Channel 13/1(In1)
  Decode Channel 1/1(Out1) -> Scope 8/1  "IO682_SerialIN_CH1"
  Decode Channel 2/1(Out1) -> Scope 8/2  "IO682_SerialIN_CH2"
  Decode Channel 13/1(Out1) -> Scope 11/1  "IO682_SerialIN_CH13"
  Decode Channel 6/1(Out1) -> Scope 9/2  "IO682_SerialIN_CH6"
  Receive v2 1/1 -> Decode Channel 2/1(In1)
  Encode Channel 8/1(Out1) -> Send v2 7/1
  Receive v2 5/1 -> Decode Channel 6/1(In1)
  Receive v2 4/1 -> Decode Channel 5/1(In1)
  Decode Channel 7/1(Out1) -> Scope 5/1  "IO682_SerialIN_CH7"
  Encode Channel 5/1(Out1) -> Send v2 4/1
  Receive v2 6/1 -> Decode Channel 7/1(In1)
  Decode Channel 4/1(Out1) -> Scope 4/2  "IO682_SerialIN_CH4"
  Encode Channel 3/1(Out1) -> Send v2 2/1
  Encode Channel 12/1(Out1) -> Send v2 11/1

== system speedgoat_test_SN5659_R2021b/IO941-SPDT-64 ==
  Data Type Conversion : DataTypeConversion
  Pulse Generator : DiscretePulseGenerator  Period=1000  PulseWidth=500  SampleTime=Ts_IO941
  "Relays " : speedgoatlib_PIL/Relays   id=1  card_type=IO941-SPDT-64 (64 SPDT Ruthenium Reed Relays)  channel_vector=[1,10,20,30,40,50,60,64]  init_vector=[0]  reset_vector=[0]  vector_ports=off  show_output=on  ts=Ts_IO941  slot=-1  NumCh=64  DeviceID=0  SubDeviceID=0  AltDeviceID=0  AltSubDeviceID=0  VendorID=0  SubVendorID=0  disable_settling_time=off
      settings: SourceProductName=Simulink Real-Time: Speedgoat I/O Driver Library
  "Scope  " : Scope  NumInputPorts=8
  wires:
  Pulse Generator/1 -> Data Type Conversion/1
  Data Type Conversion/1 -> "Relays "/1, "Relays "/8, "Relays "/7, "Relays "/6, "Relays "/5, "Relays "/4, "Relays "/3, "Relays "/2
  "Relays "/1 -> "Scope  "/1  "IO941_CH1"
  "Relays "/2 -> "Scope  "/2  "IO941_CH2"
  "Relays "/3 -> "Scope  "/3  "IO941_CH3"
  "Relays "/4 -> "Scope  "/4  "IO941_CH4"
  "Relays "/8 -> "Scope  "/8  "IO941_CH8"
  "Relays "/7 -> "Scope  "/7  "IO941_CH7"
  "Relays "/5 -> "Scope  "/5  "IO941_CH5"
  "Relays "/6 -> "Scope  "/6  "IO941_CH6"

== system speedgoat_test_SN5659_R2021b/IO612/CAN Read Loop - Port 3 ==
  SampleTime : Inport
  CAN Read : speedgoatlib_IO612/CAN Read  id=1  sampleTime=-1  portSelection=2  messageType=CAN  BusOutput=off  protl=IO612  ptIdx=1  isFDMod=0
      settings: SourceProductName=Simulink Real-Time: Speedgoat Library
  CAN Unpack : canmsglib/CAN Unpack  MsgList=(none)  MsgName=CAN Msg  MsgIDType=Standard (11-bit identifier)  MsgIdentifier=100  MsgLength=8  SignalInfo={'Signal1','0','64','LE','double','Standard','0','1','0','-Inf','Inf'}  IDPort=off  TimestampPort=off  ErrorPort=off  RemotePort=off  LengthPort=off  StatusPort=off  ApplyMinMax=off
      settings: SourceProductBaseCode=ME,XP,VN
  CAN Unpack1 : canmsglib/CAN Unpack  MsgList=(none)  MsgName=CAN Msg  MsgIDType=Standard (11-bit identifier)  MsgIdentifier=101  MsgLength=8  SignalInfo={'Signal1','0','64','LE','double','Standard','0','1','0','-Inf','Inf'}  IDPort=off  TimestampPort=off  ErrorPort=off  RemotePort=off  LengthPort=off  StatusPort=off  ApplyMinMax=off
      settings: SourceProductBaseCode=ME,XP,VN
  CAN Unpack2 : canmsglib/CAN Unpack  MsgList=(none)  MsgName=CAN Msg  MsgIDType=Standard (11-bit identifier)  MsgIdentifier=102  MsgLength=8  SignalInfo={'Signal1','0','64','LE','double','Standard','0','1','0','-Inf','Inf'}  IDPort=off  TimestampPort=off  ErrorPort=off  RemotePort=off  LengthPort=off  StatusPort=off  ApplyMinMax=off
      settings: SourceProductBaseCode=ME,XP,VN
  Terminator : Terminator
  While Iterator : WhileIterator  MaxIters=501  WhileBlockType=do-while
  ID100_Signal1 : Outport
  ID101_Signal1 : Outport  Port=2
  ID102_Signal1 : Outport  Port=3
  wires:
  SampleTime/1 -> Terminator/1
  CAN Unpack2/1 -> ID102_Signal1/1
  CAN Unpack1/1 -> ID101_Signal1/1
  CAN Unpack/1 -> ID100_Signal1/1
  CAN Read/1 -> While Iterator/1
  CAN Read/2 -> CAN Unpack/1, CAN Unpack1/1, CAN Unpack2/1

== system speedgoat_test_SN5659_R2021b/IO612/CAN Read Loop - Port 4 ==
  SampleTime : Inport
  CAN Read1 : speedgoatlib_IO612/CAN Read  id=1  sampleTime=-1  portSelection=4  messageType=CAN  BusOutput=off  protl=IO612  ptIdx=3  isFDMod=0
      settings: SourceProductName=Simulink Real-Time: Speedgoat Library
  CAN Unpack : canmsglib/CAN Unpack  MsgList=(none)  MsgName=CAN Msg  MsgIDType=Standard (11-bit identifier)  MsgIdentifier=300  MsgLength=8  SignalInfo={'Signal1','0','64','LE','double','Standard','0','1','0','-Inf','Inf'}  IDPort=off  TimestampPort=off  ErrorPort=off  RemotePort=off  LengthPort=off  StatusPort=off  ApplyMinMax=off
      settings: SourceProductBaseCode=ME,XP,VN
  CAN Unpack1 : canmsglib/CAN Unpack  MsgList=(none)  MsgName=CAN Msg  MsgIDType=Standard (11-bit identifier)  MsgIdentifier=301  MsgLength=8  SignalInfo={'Signal1','0','64','LE','double','Standard','0','1','0','-Inf','Inf'}  IDPort=off  TimestampPort=off  ErrorPort=off  RemotePort=off  LengthPort=off  StatusPort=off  ApplyMinMax=off
      settings: SourceProductBaseCode=ME,XP,VN
  CAN Unpack2 : canmsglib/CAN Unpack  MsgList=(none)  MsgName=CAN Msg  MsgIDType=Standard (11-bit identifier)  MsgIdentifier=302  MsgLength=8  SignalInfo={'Signal1','0','64','LE','double','Standard','0','1','0','-Inf','Inf'}  IDPort=off  TimestampPort=off  ErrorPort=off  RemotePort=off  LengthPort=off  StatusPort=off  ApplyMinMax=off
      settings: SourceProductBaseCode=ME,XP,VN
  Terminator : Terminator
  While Iterator : WhileIterator  MaxIters=501  WhileBlockType=do-while
  ID100_Signal1 : Outport
  ID101_Signal1 : Outport  Port=2
  ID102_Signal1 : Outport  Port=3
  wires:
  CAN Read1/2 -> CAN Unpack2/1, CAN Unpack1/1, CAN Unpack/1
  CAN Read1/1 -> While Iterator/1
  CAN Unpack/1 -> ID100_Signal1/1
  CAN Unpack1/1 -> ID101_Signal1/1
  CAN Unpack2/1 -> ID102_Signal1/1
  SampleTime/1 -> Terminator/1

== system speedgoat_test_SN5659_R2021b/IO682/Decode Channel 1 ==
  note: Because of the limited number of bits
      | that are encoded and sent by ARINC,
      | these values may differ from values
      | on the input side.
  In1 : Inport
  Decode 1 : speedgoatlib_IO682/Decode v2   parMode=Standard  parLabel=100  parDataType=[1]  parResolution=[1024]  parSyncMask=hex2dec('0x0')  parSyncValue=hex2dec('0x0')  parCustomDataType=Raw  parDataLSB=9  parDataMSB=31  parBitPosition=[9, 31]  parScaleBNR=1  parExponent=8  parMantissa=14  parTimeTags=off  parHoldLastVal=on  parStatus=off
      settings: SourceProductName=Simulink Real-Time: Speedgoat I/O Blockset
  Decode 3 : speedgoatlib_IO682/Decode v2   parMode=Standard  parLabel=102  parDataType=[1]  parResolution=[65536]  parSyncMask=hex2dec('0x0')  parSyncValue=hex2dec('0x0')  parCustomDataType=Raw  parDataLSB=9  parDataMSB=31  parBitPosition=[9, 31]  parScaleBNR=1  parExponent=8  parMantissa=14  parTimeTags=off  parHoldLastVal=on  parStatus=off
      settings: SourceProductName=Simulink Real-Time: Speedgoat I/O Blockset
  Decode 4 : speedgoatlib_IO682/Decode v2   parMode=Standard  parLabel=103  parDataType=[1]  parResolution=[1024]  parSyncMask=hex2dec('0x0')  parSyncValue=hex2dec('0x0')  parCustomDataType=Raw  parDataLSB=9  parDataMSB=31  parBitPosition=[9, 31]  parScaleBNR=1  parExponent=8  parMantissa=14  parTimeTags=off  parHoldLastVal=on  parStatus=off
      settings: SourceProductName=Simulink Real-Time: Speedgoat I/O Blockset
  Decode 5 : speedgoatlib_IO682/Decode v2   parMode=Standard  parLabel=101  parDataType=[2]  parResolution=[.1]  parSyncMask=hex2dec('0x0')  parSyncValue=hex2dec('0x0')  parCustomDataType=Raw  parDataLSB=9  parDataMSB=31  parBitPosition=[9, 31]  parScaleBNR=1  parExponent=8  parMantissa=14  parTimeTags=off  parHoldLastVal=on  parStatus=off
      settings: SourceProductName=Simulink Real-Time: Speedgoat I/O Blockset
  Mux : Mux
  Out1 : Outport
  wires:
  In1/1 -> Decode 3/1, Decode 4/1, Decode 5/1, Decode 1/1
  Mux/1 -> Out1/1
  Decode 5/1 -> Mux/2
  Decode 1/1 -> Mux/1
  Decode 3/1 -> Mux/3
  Decode 4/1 -> Mux/4

== system speedgoat_test_SN5659_R2021b/IO682/Decode Channel 10 ==
  In1 : Inport
  Decode 1 : speedgoatlib_IO682/Decode v2   parMode=Standard  parLabel=100  parDataType=[1]  parResolution=[1024]  parSyncMask=hex2dec('0x0')  parSyncValue=hex2dec('0x0')  parCustomDataType=Raw  parDataLSB=9  parDataMSB=31  parBitPosition=[9, 31]  parScaleBNR=1  parExponent=8  parMantissa=14  parTimeTags=off  parHoldLastVal=on  parStatus=off
      settings: SourceProductName=Simulink Real-Time: Speedgoat I/O Blockset
  Decode 2 : speedgoatlib_IO682/Decode v2   parMode=Standard  parLabel=101  parDataType=[2]  parResolution=[.1]  parSyncMask=hex2dec('0x0')  parSyncValue=hex2dec('0x0')  parCustomDataType=Raw  parDataLSB=9  parDataMSB=31  parBitPosition=[9, 31]  parScaleBNR=1  parExponent=8  parMantissa=14  parTimeTags=off  parHoldLastVal=on  parStatus=off
      settings: SourceProductName=Simulink Real-Time: Speedgoat I/O Blockset
  Decode 3 : speedgoatlib_IO682/Decode v2   parMode=Standard  parLabel=102  parDataType=[1]  parResolution=[65536]  parSyncMask=hex2dec('0x0')  parSyncValue=hex2dec('0x0')  parCustomDataType=Raw  parDataLSB=9  parDataMSB=31  parBitPosition=[9, 31]  parScaleBNR=1  parExponent=8  parMantissa=14  parTimeTags=off  parHoldLastVal=on  parStatus=off
      settings: SourceProductName=Simulink Real-Time: Speedgoat I/O Blockset
  Decode 4 : speedgoatlib_IO682/Decode v2   parMode=Standard  parLabel=103  parDataType=[1]  parResolution=[1024]  parSyncMask=hex2dec('0x0')  parSyncValue=hex2dec('0x0')  parCustomDataType=Raw  parDataLSB=9  parDataMSB=31  parBitPosition=[9, 31]  parScaleBNR=1  parExponent=8  parMantissa=14  parTimeTags=off  parHoldLastVal=on  parStatus=off
      settings: SourceProductName=Simulink Real-Time: Speedgoat I/O Blockset
  Mux : Mux
  Out1 : Outport
  wires:
  Decode 1/1 -> Mux/1
  In1/1 -> Decode 4/1, Decode 3/1, Decode 2/1, Decode 1/1
  Mux/1 -> Out1/1
  Decode 4/1 -> Mux/4
  Decode 3/1 -> Mux/3
  Decode 2/1 -> Mux/2

== system speedgoat_test_SN5659_R2021b/IO682/Decode Channel 11 ==
  In1 : Inport
  Decode 1 : speedgoatlib_IO682/Decode v2   parMode=Standard  parLabel=100  parDataType=[1]  parResolution=[1024]  parSyncMask=hex2dec('0x0')  parSyncValue=hex2dec('0x0')  parCustomDataType=Raw  parDataLSB=9  parDataMSB=31  parBitPosition=[9, 31]  parScaleBNR=1  parExponent=8  parMantissa=14  parTimeTags=off  parHoldLastVal=on  parStatus=off
      settings: SourceProductName=Simulink Real-Time: Speedgoat I/O Blockset
  Decode 2 : speedgoatlib_IO682/Decode v2   parMode=Standard  parLabel=101  parDataType=[2]  parResolution=[.1]  parSyncMask=hex2dec('0x0')  parSyncValue=hex2dec('0x0')  parCustomDataType=Raw  parDataLSB=9  parDataMSB=31  parBitPosition=[9, 31]  parScaleBNR=1  parExponent=8  parMantissa=14  parTimeTags=off  parHoldLastVal=on  parStatus=off
      settings: SourceProductName=Simulink Real-Time: Speedgoat I/O Blockset
  Decode 3 : speedgoatlib_IO682/Decode v2   parMode=Standard  parLabel=102  parDataType=[1]  parResolution=[65536]  parSyncMask=hex2dec('0x0')  parSyncValue=hex2dec('0x0')  parCustomDataType=Raw  parDataLSB=9  parDataMSB=31  parBitPosition=[9, 31]  parScaleBNR=1  parExponent=8  parMantissa=14  parTimeTags=off  parHoldLastVal=on  parStatus=off
      settings: SourceProductName=Simulink Real-Time: Speedgoat I/O Blockset
  Decode 4 : speedgoatlib_IO682/Decode v2   parMode=Standard  parLabel=103  parDataType=[1]  parResolution=[1024]  parSyncMask=hex2dec('0x0')  parSyncValue=hex2dec('0x0')  parCustomDataType=Raw  parDataLSB=9  parDataMSB=31  parBitPosition=[9, 31]  parScaleBNR=1  parExponent=8  parMantissa=14  parTimeTags=off  parHoldLastVal=on  parStatus=off
      settings: SourceProductName=Simulink Real-Time: Speedgoat I/O Blockset
  Mux : Mux
  Out1 : Outport
  wires:
  Decode 1/1 -> Mux/1
  Decode 2/1 -> Mux/2
  Decode 4/1 -> Mux/4
  Decode 3/1 -> Mux/3
  Mux/1 -> Out1/1
  In1/1 -> Decode 4/1, Decode 3/1, Decode 2/1, Decode 1/1
